simulink model "RealTimeSimulation"  (R2024b)
settings: Solver=ode3  StartTime=0.0  StopTime=10.0  FixedStep=0.001  RelTol=1e-3
InitFcn:
  | Init
values from neighbouring files (symbols this model uses):
  degs2rpm = 60/360    (= 0.166666666667)    [Init.m]    (also in ModelParams.m; load_params_inertial_case.m)
  delta_est = 1/sqrt(2)    [Init.m]    (also in code.m; main.m)
  Kd = Kp * Td    [Init.m]    (also in code.m; main.m)
  Ki = Kp / Ti    [Init.m]    (also in code.m; main.m)
  Kp = deltak * cos(deltaphi)    [Init.m]    (also in code.m = deltak*cos(deltaphi); main.m = deltak*cos(deltaphi))
  rpm2degs = 360/60    (= 6)    [Init.m]    (also in ModelParams.m; load_params_inertial_case.m)
  rpm2rads = 2*pi/60    (= 0.10471975512)    [Init.m]    (also in ModelParams.m; load_params_inertial_case.m)
  tl = 1/(3*wgc)    [Init.m]    (also in code.m = 1/cut_off; main.m = 1/cut_off)
  wc = 2*pi*20    (= 125.663706144)    [Init.m]    (also in code.m; main.m)
undefined symbols (not defined in the file or in its folder): gbox, mld, mot, sens
settings Model: Creator=Banaan  LastModifiedBy=Banaan

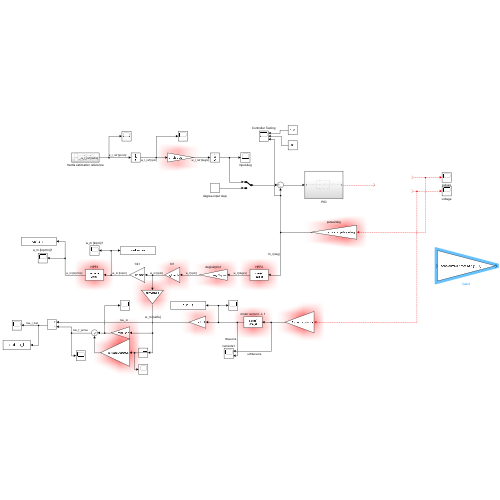
[thumbnail: Simulink's stored preview of the top-level diagram]
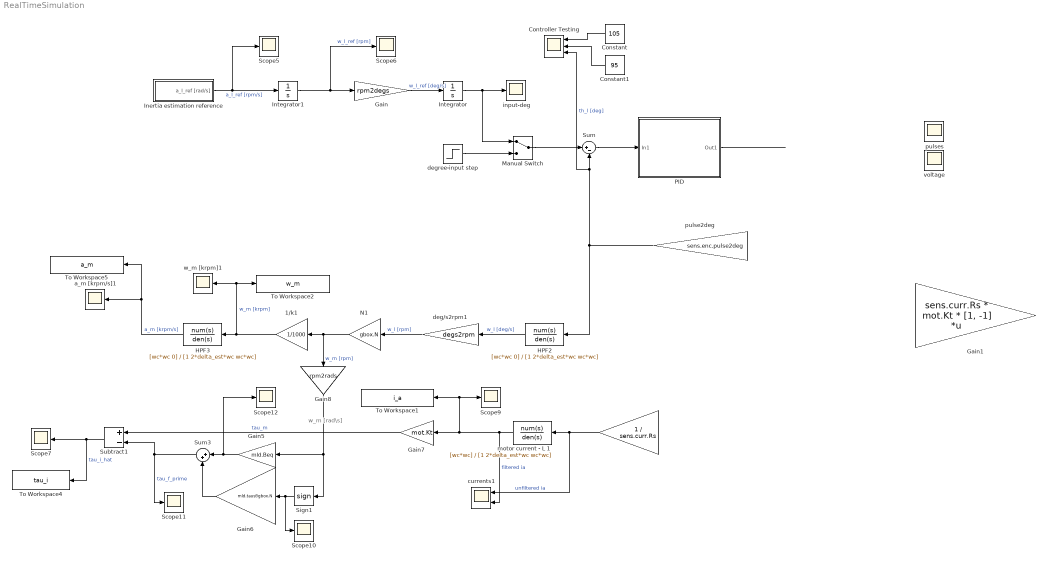
== system RealTimeSimulation ==
  note: w_m [rad\s]
  " " : Gain  Gain=1 / sens.curr.Rs
  1/k1 : Gain  Gain=1/1000
  Constant : Constant  Value=105
  Constant1 : Constant  Value=95
  Controller Testing : Scope  NumInputPorts=3
  Gain : Gain  Gain=rpm2degs
  Gain1 : Gain  Gain=sens.curr.Rs * mot.Kt * [1, -1]  Multiplication=Matrix(K*u)
  Gain5 : Gain  Gain=mld.Beq
  Gain6 : Gain  Gain=mld.tausf/gbox.N
  Gain7 : Gain  Gain=mot.Kt
  Gain8 : Gain  Gain=rpm2rads
  HPF2 : TransferFcn  Numerator=[wc*wc 0]  Denominator=[1 2*delta_est*wc wc*wc]
  HPF3 : TransferFcn  Numerator=[wc*wc 0]  Denominator=[1 2*delta_est*wc wc*wc]
  Inertia estimation reference : Subsystem
  Integrator : Integrator
  Integrator1 : Integrator
  Manual Switch : ManualSwitch
  N1 : Gain  Gain=gbox.N
  PID : Subsystem
  Scope{5..7,9..12} (7 alike) : Scope
  Sign1 : Signum  ZeroCross=off
  Subtract1 : Sum  Inputs=+-
  Sum : Sum  Inputs=|+-
  Sum3 : Sum  Inputs=|++
  To Workspace1 : ToWorkspace  VariableName=i_a  SaveFormat=Structure With Time  SampleTime=-1
  To Workspace2 : ToWorkspace  VariableName=w_m  SaveFormat=Structure With Time  SampleTime=-1
  To Workspace4 : ToWorkspace  VariableName=tau_i  SaveFormat=Structure With Time  SampleTime=-1
  To Workspace5 : ToWorkspace  VariableName=a_m  SaveFormat=Structure With Time  SampleTime=-1
  a_m [krpm/s]1 : Scope
  currents1 : Scope  NumInputPorts=2
  deg/s2rpm1 : Gain  Gain=degs2rpm
  degree-input step : Step  Time=0  After=100  SampleTime=0
  input-deg : Scope
  motor current - L 1 : TransferFcn  Numerator=[wc*wc]  Denominator=[1 2*delta_est*wc wc*wc]
  pulse2deg : Gain  Gain=sens.enc.pulse2deg
  pulses : Scope
  voltage : Scope
  w_m [krpm]1 : Scope
  wires:
  Gain8/1 -> Sign1/1, Gain5/1
  N1/1 -> Gain8/1, 1/k1/1  "w_m [rpm]"
  HPF3/1 -> a_m [krpm/s]1/1, To Workspace5/1  "a_m [krpm/s]"
  Integrator/1 -> Manual Switch/1, input-deg/1
  Sign1/1 -> Scope10/1, Gain6/1
  " "/1 -> currents1/1, motor current - L 1/1  "unfiltered ia"
  motor current - L 1/1 -> To Workspace1/1, Scope9/1, Gain7/1, currents1/2  "filtered ia"
  HPF2/1 -> deg/s2rpm1/1  "w_l [deg/s]"
  Gain6/1 -> Sum3/2
  Gain5/1 -> Sum3/1, Scope12/1
  Gain7/1 -> Subtract1/1  "tau_m"
  Subtract1/1 -> To Workspace4/1, Scope7/1  "tau_i_hat"
  1/k1/1 -> HPF3/1, To Workspace2/1, w_m [krpm]1/1  "w_m [krpm]"
  Integrator1/1 -> Scope6/1, Gain/1  "w_l_ref [rpm]"
  PID/1(Out1) -> ?
  degree-input step/1 -> Manual Switch/2
  ? -> pulses/1, pulse2deg/1
  ? -> voltage/1, " "/1
  Inertia estimation reference/1(a_l_ref [rad/s]) -> Scope5/1, Integrator1/1  "a_l_ref [rpm/s]"
  pulse2deg/1 -> HPF2/1, Controller Testing/3, Sum/2  "th_l [deg]"
  deg/s2rpm1/1 -> N1/1  "w_l [rpm]"
  Manual Switch/1 -> Sum/1
  Sum/1 -> PID/1(In1)
  Gain/1 -> Integrator/1  "w_l_ref [deg/s]"
  Constant1/1 -> Controller Testing/2
  Sum3/1 -> Subtract1/2, Scope11/1  "tau_f_prime"
  Constant/1 -> Controller Testing/1

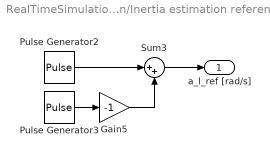
== system RealTimeSimulation/Inertia estimation reference ==
  Gain5 : Gain  Gain=-1
  Pulse Generator2 : DiscretePulseGenerator  PulseType=Time based  Amplitude=450  PulseWidth=50
  Pulse Generator3 : DiscretePulseGenerator  PulseType=Time based  Amplitude=450  PulseWidth=50  PhaseDelay=1
  Sum3 : Sum  Inputs=|++
  a_l_ref [rad/s] : Outport
  wires:
  Pulse Generator3/1 -> Gain5/1
  Pulse Generator2/1 -> Sum3/1
  Gain5/1 -> Sum3/2
  Sum3/1 -> a_l_ref [rad/s]/1

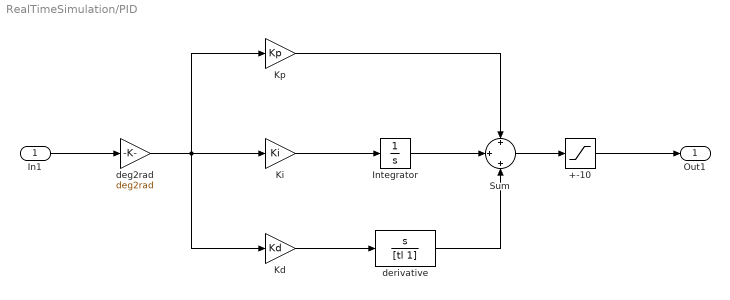
== system RealTimeSimulation/PID ==
  In1 : Inport
  +-10 : Saturate  UpperLimit=10  LowerLimit=-10
  Integrator : Integrator
  Kd : Gain  Gain=Kd
  Ki : Gain  Gain=Ki
  Kp : Gain  Gain=Kp
  Sum : Sum  Inputs=+|+|+
  deg2rad : Gain  Gain=deg2rad
  derivative : TransferFcn  Numerator=[1 0]  Denominator=[tl 1]
  Out1 : Outport
  wires:
  In1/1 -> deg2rad/1
  deg2rad/1 -> Kd/1, Kp/1, Ki/1
  Ki/1 -> Integrator/1
  Kp/1 -> Sum/1
  Integrator/1 -> Sum/2
  Kd/1 -> derivative/1
  derivative/1 -> Sum/3
  Sum/1 -> +-10/1
  +-10/1 -> Out1/1
